simulink model "model"  (R2015a)
settings: Solver=ode45  StartTime=0.0  StopTime=10.0  RelTol=1e-3
PreLoadFcn:
  | init
values from neighbouring files (symbols this model uses):
  g = -9.81    [init.m]
  m = 0.5    [init.m]
undefined symbols (not defined in the file or in its folder): a, b
settings Model: Creator=Felipe Vargas  LastModifiedBy=Felipe Vargas

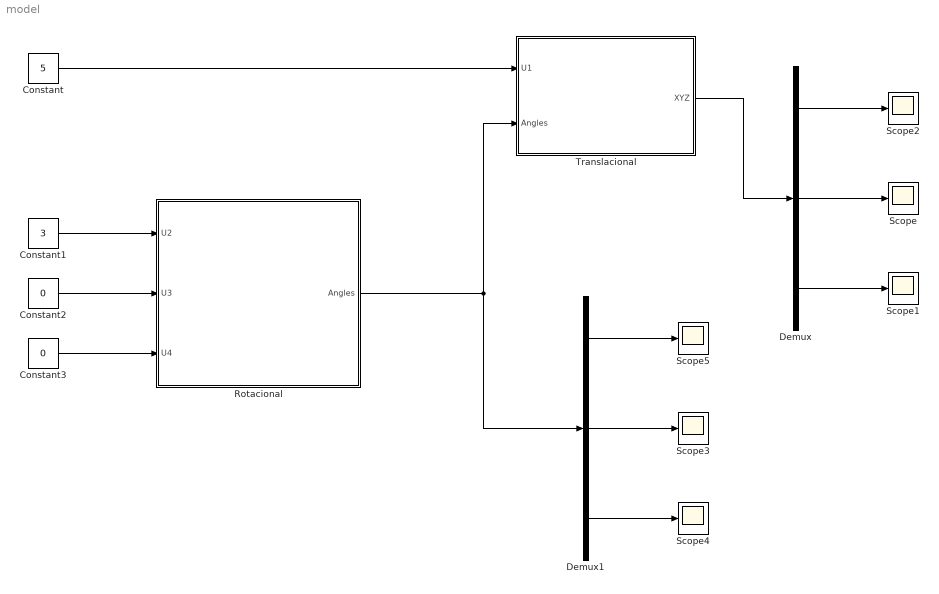
== system model ==
  Constant : Constant  Value=5
  Constant1 : Constant  Value=3
  Constant2 : Constant  Value=0
  Constant3 : Constant  Value=0
  Demux : Demux  Outputs=3
  Demux1 : Demux  Outputs=3
  "Rotacional " : Subsystem
  Scope{,1..5} (6 alike) : Scope
      Scope2 settings: SaveName=ScopeData2
      Scope3 settings: SaveName=ScopeData3
      Scope4 settings: SaveName=ScopeData4
      Scope5 settings: SaveName=ScopeData5
  Translacional : Subsystem
  wires:
  "Rotacional "/1(Angles) -> Translacional/2(Angles), Demux1/1
  Demux/1 -> Scope2/1
  Demux/2 -> Scope/1
  Demux/3 -> Scope1/1
  Demux1/1 -> Scope5/1
  Demux1/2 -> Scope3/1
  Demux1/3 -> Scope4/1
  Translacional/1(XYZ) -> Demux/1
  Constant1/1 -> "Rotacional "/1(U2)
  Constant2/1 -> "Rotacional "/2(U3)
  Constant3/1 -> "Rotacional "/3(U4)
  Constant/1 -> Translacional/1(U1)

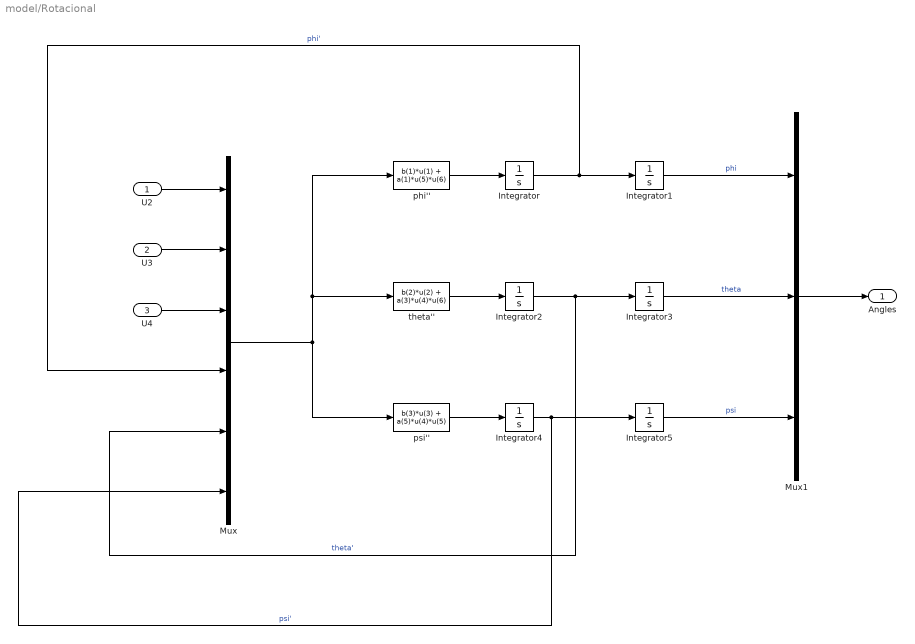
== system model/Rotacional  ==
  U2 : Inport
  U3 : Inport  Port=2
  U4 : Inport  Port=3
  Integrator{,1..5} (6 alike) : Integrator
  Mux : Mux  Inputs=6
  Mux1 : Mux  Inputs=3
  phi'' : Fcn  Expr=b(1)*u(1) + a(1)*u(5)*u(6)
  psi'' : Fcn  Expr=b(3)*u(3) + a(5)*u(4)*u(5)
  theta'' : Fcn  Expr=b(2)*u(2) + a(3)*u(4)*u(6)
  Angles : Outport
  wires:
  U2/1 -> Mux/1
  U3/1 -> Mux/2
  U4/1 -> Mux/3
  phi''/1 -> Integrator/1
  Integrator/1 -> Mux/4, Integrator1/1  "phi'"
  Mux/1 -> psi''/1, theta''/1, phi''/1
  theta''/1 -> Integrator2/1
  Integrator2/1 -> Mux/5, Integrator3/1  "theta'"
  psi''/1 -> Integrator4/1
  Integrator4/1 -> Mux/6, Integrator5/1  "psi'"
  Integrator1/1 -> Mux1/1  "phi"
  Integrator3/1 -> Mux1/2  "theta"
  Mux1/1 -> Angles/1
  Integrator5/1 -> Mux1/3  "psi"

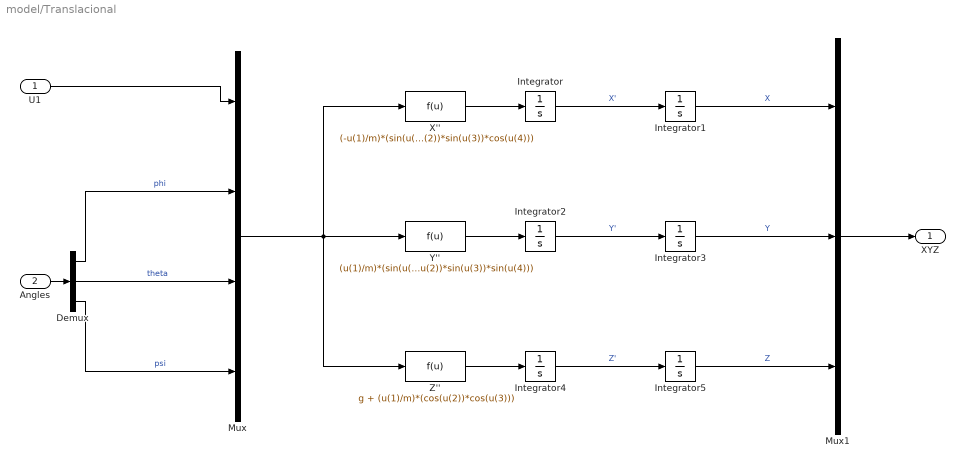
== system model/Translacional ==
  U1 : Inport
  Angles : Inport  Port=2
  Demux : Demux  Outputs=3
  Integrator{,1..5} (6 alike) : Integrator
  Mux : Mux
  Mux1 : Mux  Inputs=3
  X'' : Fcn  Expr=(-u(1)/m)*(sin(u(2))*sin(u(4)) + cos(u(2))*sin(u(3))*cos(u(4)))
  Y'' : Fcn  Expr=(u(1)/m)*(sin(u(2))*cos(u(4)) - cos(u(2))*sin(u(3))*sin(u(4)))
  Z'' : Fcn  Expr=g + (u(1)/m)*(cos(u(2))*cos(u(3)))
  XYZ : Outport
  wires:
  X''/1 -> Integrator/1
  Integrator/1 -> Integrator1/1  "X'"
  Integrator1/1 -> Mux1/1  "X"
  Mux1/1 -> XYZ/1
  Angles/1 -> Demux/1
  Mux/1 -> Z''/1, Y''/1, X''/1
  U1/1 -> Mux/1
  Demux/1 -> Mux/2  "phi"
  Demux/2 -> Mux/3  "theta"
  Demux/3 -> Mux/4  "psi"
  Y''/1 -> Integrator2/1
  Integrator2/1 -> Integrator3/1  "Y'"
  Integrator3/1 -> Mux1/2  "Y"
  Z''/1 -> Integrator4/1
  Integrator4/1 -> Integrator5/1  "Z'"
  Integrator5/1 -> Mux1/3  "Z"
